simulink model "NeuromuscularModelwReflex2"  (R2019b)
settings: Solver=ode15s  StartTime=0.0  StopTime=30  MaxStep=.01  RelTol=1e-4  AbsTol=1e-6  EnableMultiTasking=on
values from neighbouring files (symbols this model uses):
  dt_visual = 1/30    (= 0.0333333333333)    [evaluateCost.m]    (also in optimize.m)
  LceOffsetTA = 1-0.5*w    [ControlParams.m]
  legAngleTgt = 1.2    [ControlParams.m]    (also in assignGains_novirtmuscle.m = Gains(38))
  LlegLengthClr = .9    (= 0.9)    [ControlParams.m]    (also in assignGains.m = Gains(39); assignGains_novirtmuscle.m = Gains(20))
  LongDelay = 0.020    (= 0.02)    [ControlParams.m]
  MidDelay = 0.010    (= 0.01)    [ControlParams.m]
  RlegLengthClr = .9    (= 0.9)    [ControlParams.m]    (also in assignGains.m = Gains(83); assignGains_novirtmuscle.m = Gains(34))
  ShortDelay = 0.005    [ControlParams.m]
  simbiconGainD = 5*pi/180    (= 0.0872664625997)    [ControlParams.m]    (also in assignGains_novirtmuscle.m = Gains(35))
  simbiconGainV = 5*pi/180    (= 0.0872664625997)    [ControlParams.m]    (also in assignGains_novirtmuscle.m = Gains(36))
  simbiconLegAngle0 = 85*pi/180    (= 1.4835298642)    [ControlParams.m]    (also in assignGains_novirtmuscle.m = Gains(37))
  termination_height = 0.5    [ControlParams.m]
undefined symbols (not defined in the file or in its folder): footCenterToCGDist, footInertia, footMass, g, loptGAS, loptHAM, loptHAMCut, loptTA, lslackGAS, lslackHAM, lslackHAMCut, phimaxGASa, phimaxGASk, phimaxHAMk, phirefGASa, phirefGASk, phirefHAMh, phirefHAMk, rGASa, rGASk, rHAMh, rHAMk, rhoGASa, rhoGASk, rhoHAMh, rhoHAMk, X, Y, Z
libraries: NeuroMuscularLibrary x88, sm_lib x22, nesl_utility x20, simulink x6, simulink_extras x2
(part 2 of 3)

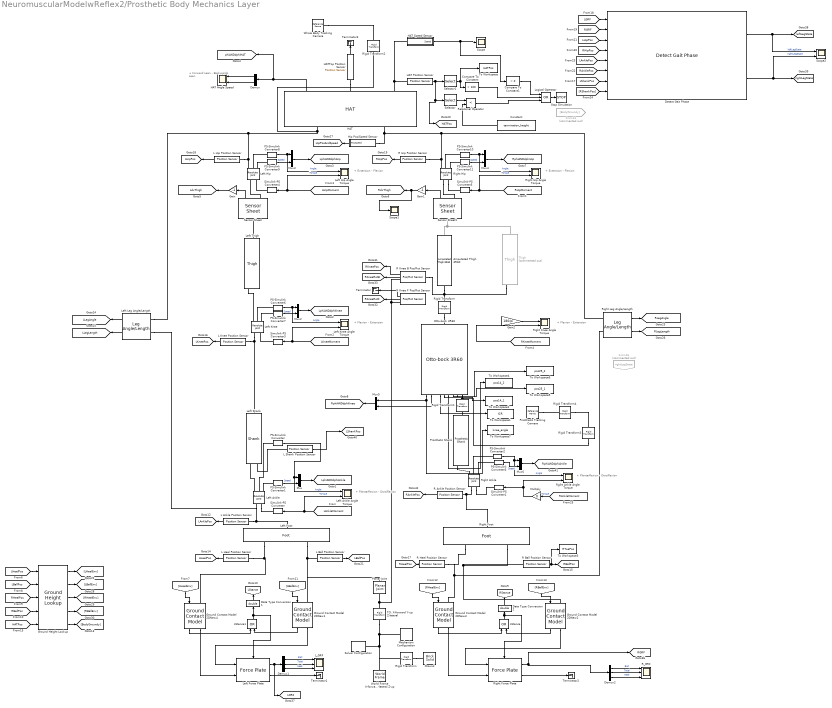
== system NeuromuscularModelwReflex2/Prosthetic Body Mechanics Layer ==
  note: + Plantarflexion
      | -  Dorsiflexion
  note: + Flexion
      | -  Extension
  note: + Extension
      | -  Flexion
  note: + Forward Lean
      | -  Backwards Lean
  note: + Extension
      | -  Flexion
  note: + Flexion
      | -  Extension
  note: + Plantarflexion
      | -  Dorsiflexion
  Amputated Thigh 3R60 : NeuroMuscularLibrary/Amputated Thigh 3R60  SystemSampleTime=-1  Latency=0  AutoFrameSizeCalculation=off
  Compare To Constant : simulink/Logic and Bit Operations/Compare To Constant  relop=>  const=100  OutDataTypeStr=boolean
  Compare To Constant1 : simulink/Logic and Bit Operations/Compare To Constant  relop=<  const=0  OutDataTypeStr=boolean
  Constant : Constant  Value=termination_height
  Data Type Conversion1 : DataTypeConversion  OutDataTypeStr=double
  Data Type Conversion2 : DataTypeConversion  OutDataTypeStr=double
  Demux : Demux  Outputs=2
  Demux1 : Demux  Outputs=3
  Demux2 : Demux  Outputs=3
  Detect Gait Phase : NeuroMuscularLibrary/Detect Gait Phase  SystemSampleTime=-1  Latency=0  AutoFrameSizeCalculation=off
  From14 : From  Commented=on  GotoTag=BodyGroundy
  From16 : From  Commented=on  GotoTag=rightLegState  TagVisibility=global
  Gain : Gain  Gain=-1
  Gain1 : Gain  Gain=-1
  Gain2 : Gain  Gain=180/pi
  Ground : sm_lib/Body Elements/Brick Solid  GraphicAmbientColor=[0.15 0.15 0.15 1.0]  BasedOnType=Density  BrickDimensions=[3 1 .01]  BrickDimensionUnits=m  CenterOfMass=[-footCenterToCGDist 0 0]  CenterOfMassUnits=m  GraphicDiffuseColor=[0.4 0.2 0.0]  Density=1000  DensityUnits=kg/(m^3)  DoExposeReferenceFrame=on  GraphicEmissiveColor=[0.0 0.0 0.0 1.0]  ExportEntireGeometry=off  SerializedFrames=<Frames/>  MarkerShape=Sphere  MarkerSize=10  GraphicType=FromGeometry  InertiaType=CalculateFromGeometry  Mass=footMass  MassUnits=kg  MomentsOfInertia=[0 0 footInertia]  MomentsOfInertiaUnits=kg*m^2  GraphicOpacity=1.0  ProductsOfInertia=[0 0 0]  ProductsOfInertiaUnits=kg*m^2  GraphicShininess=75  GraphicSpecularColor=[0.5 0.5 0.5 1.0]  GraphicVisPropType=SimpleVisualProperties
  Ground Contact Model 2DNew{1..4} (4 alike) : NeuroMuscularLibrary/Ground Contact Model  SystemSampleTime=-1  Latency=0  AutoFrameSizeCalculation=off
  Ground Height Lookup : NeuroMuscularLibrary/Ground Height Lookup  SystemSampleTime=-1  Latency=0  AutoFrameSizeCalculation=off
  HAT : NeuroMuscularLibrary/HAT  SystemSampleTime=-1  Latency=0  AutoFrameSizeCalculation=off
  HAT Position Sensor : NeuroMuscularLibrary/Position Sensor  SystemSampleTime=-1  Latency=0  AutoFrameSizeCalculation=off
  HAT Angle Speed : Scope  NumInputPorts=2
  HAT Speed Sensor : Subsystem
  HATTop Position Sensor : NeuroMuscularLibrary/Position Sensor  SystemSampleTime=-1  Latency=0  AutoFrameSizeCalculation=off
  Hip Pos/Speed Sensor : Subsystem
  L Ankle Position Sensor : NeuroMuscularLibrary/Position Sensor  SystemSampleTime=-1  Latency=0  AutoFrameSizeCalculation=off
  L Ball Position Sensor : NeuroMuscularLibrary/Position Sensor  SystemSampleTime=-1  Latency=0  AutoFrameSizeCalculation=off
  L Heel Position Sensor : NeuroMuscularLibrary/Position Sensor  SystemSampleTime=-1  Latency=0  AutoFrameSizeCalculation=off
  L Hip Position Sensor : NeuroMuscularLibrary/Position Sensor  SystemSampleTime=-1  Latency=0  AutoFrameSizeCalculation=off
  L Knee Position Sensor : NeuroMuscularLibrary/Position Sensor  SystemSampleTime=-1  Latency=0  AutoFrameSizeCalculation=off
  L Shank Position Sensor : NeuroMuscularLibrary/Position Sensor  SystemSampleTime=-1  Latency=0  AutoFrameSizeCalculation=off
  LStance : Logic  Operator=OR  AllPortsSameDT=off  OutDataTypeStr=boolean
  LStance1 : Logic  Operator=OR  AllPortsSameDT=off  OutDataTypeStr=boolean
  L_GRF : Scope  NumInputPorts=3
  Left Ankle : sm_lib/Joints/Revolute Joint  JointMode=Normal  SenseConstraintForce=off  SenseConstraintForceX=off  SenseConstraintForceY=off  SenseConstraintForceZ=off  SenseConstraintTorque=off  SenseConstraintTorqueX=off  SenseConstraintTorqueY=off  SenseConstraintTorqueZ=off  SenseTotalForce=off  SenseTotalForceX=off  SenseTotalForceY=off  SenseTotalForceZ=off  SenseTotalTorque=off  SenseTotalTorqueX=off  SenseTotalTorqueY=off  SenseTotalTorqueZ=off  CompositeWrenchDir=FollowerOnBase  CompositeWrenchFrame=BaseFrame  EquilibriumPosition=0  EquilibriumPositionUnits=deg  SpringStiffness=0  SpringStiffnessUnits=N*m/deg  DampingCoefficient=0  DampingCoefficientUnits=N*m/(deg/s)  TorqueActuationMode=InputTorque  MotionActuationMode=ComputedMotion  SensePosition=on  SenseVelocity=on  SenseAcceleration=off  SenseTorqueForce=off  SenseLowerLimitTorqueForce=off  SenseUpperLimitTorqueForce=off  LowerLimitSpecify=off  LowerLimitBound=-90  LowerLimitBoundUnits=deg  LowerLimitStiffness=1e4  LowerLimitStiffnessUnits=N*m/deg  LowerLimitDamping=10  LowerLimitDampingUnits=N*m/(deg/s)  LowerLimitTransitionRegionWidth=0.1  LowerLimitTransitionRegionWidthUnits=deg  UpperLimitSpecify=off  UpperLimitBound=90  UpperLimitBoundUnits=deg  UpperLimitStiffness=1e4  UpperLimitStiffnessUnits=N*m/deg  UpperLimitDamping=10  UpperLimitDampingUnits=N*m/(deg/s)  UpperLimitTransitionRegionWidth=0.1  UpperLimitTransitionRegionWidthUnits=deg  PositionTargetSpecify=on  PositionTargetPriority=High  PositionTargetValue=LphiAnkle0  PositionTargetValueUnits=rad  VelocityTargetSpecify=on  VelocityTargetPriority=Low  VelocityTargetValue=0  VelocityTargetValueUnits=rad/s
  Left Ankle Angle Torque : Scope  NumInputPorts=2
  Left Foot : NeuroMuscularLibrary/Foot  SystemSampleTime=-1  Latency=0  AutoFrameSizeCalculation=off
  Left Force Plate : NeuroMuscularLibrary/Force Plate  SystemSampleTime=-1  Latency=0  AutoFrameSizeCalculation=off
  Left Hip : sm_lib/Joints/Revolute Joint  JointMode=Normal  SenseConstraintForce=off  SenseConstraintForceX=off  SenseConstraintForceY=off  SenseConstraintForceZ=off  SenseConstraintTorque=off  SenseConstraintTorqueX=off  SenseConstraintTorqueY=off  SenseConstraintTorqueZ=off  SenseTotalForce=off  SenseTotalForceX=off  SenseTotalForceY=off  SenseTotalForceZ=off  SenseTotalTorque=off  SenseTotalTorqueX=off  SenseTotalTorqueY=off  SenseTotalTorqueZ=off  CompositeWrenchDir=FollowerOnBase  CompositeWrenchFrame=BaseFrame  EquilibriumPosition=0  EquilibriumPositionUnits=deg  SpringStiffness=0  SpringStiffnessUnits=N*m/deg  DampingCoefficient=0  DampingCoefficientUnits=N*m/(deg/s)  TorqueActuationMode=InputTorque  MotionActuationMode=ComputedMotion  SensePosition=on  SenseVelocity=on  SenseAcceleration=off  SenseTorqueForce=off  SenseLowerLimitTorqueForce=off  SenseUpperLimitTorqueForce=off  LowerLimitSpecify=off  LowerLimitBound=-90  LowerLimitBoundUnits=deg  LowerLimitStiffness=1e4  LowerLimitStiffnessUnits=N*m/deg  LowerLimitDamping=10  LowerLimitDampingUnits=N*m/(deg/s)  LowerLimitTransitionRegionWidth=0.1  LowerLimitTransitionRegionWidthUnits=deg  UpperLimitSpecify=off  UpperLimitBound=90  UpperLimitBoundUnits=deg  UpperLimitStiffness=1e4  UpperLimitStiffnessUnits=N*m/deg  UpperLimitDamping=10  UpperLimitDampingUnits=N*m/(deg/s)  UpperLimitTransitionRegionWidth=0.1  UpperLimitTransitionRegionWidthUnits=deg  PositionTargetSpecify=on  PositionTargetPriority=High  PositionTargetValue=LphiHip0  PositionTargetValueUnits=rad  VelocityTargetSpecify=on  VelocityTargetPriority=Low  VelocityTargetValue=0  VelocityTargetValueUnits=deg/s
  Left Hip Angle Torque : Scope  NumInputPorts=2
  Left Knee : sm_lib/Joints/Revolute Joint  JointMode=Normal  SenseConstraintForce=off  SenseConstraintForceX=off  SenseConstraintForceY=off  SenseConstraintForceZ=off  SenseConstraintTorque=off  SenseConstraintTorqueX=off  SenseConstraintTorqueY=off  SenseConstraintTorqueZ=off  SenseTotalForce=off  SenseTotalForceX=off  SenseTotalForceY=off  SenseTotalForceZ=off  SenseTotalTorque=off  SenseTotalTorqueX=off  SenseTotalTorqueY=off  SenseTotalTorqueZ=off  CompositeWrenchDir=FollowerOnBase  CompositeWrenchFrame=BaseFrame  EquilibriumPosition=0  EquilibriumPositionUnits=deg  SpringStiffness=0  SpringStiffnessUnits=N*m/deg  DampingCoefficient=0  DampingCoefficientUnits=N*m/(deg/s)  TorqueActuationMode=InputTorque  MotionActuationMode=ComputedMotion  SensePosition=on  SenseVelocity=on  SenseAcceleration=off  SenseTorqueForce=off  SenseLowerLimitTorqueForce=off  SenseUpperLimitTorqueForce=off  LowerLimitSpecify=off  LowerLimitBound=-90  LowerLimitBoundUnits=deg  LowerLimitStiffness=1e4  LowerLimitStiffnessUnits=N*m/deg  LowerLimitDamping=10  LowerLimitDampingUnits=N*m/(deg/s)  LowerLimitTransitionRegionWidth=0.1  LowerLimitTransitionRegionWidthUnits=deg  UpperLimitSpecify=off  UpperLimitBound=90  UpperLimitBoundUnits=deg  UpperLimitStiffness=1e4  UpperLimitStiffnessUnits=N*m/deg  UpperLimitDamping=10  UpperLimitDampingUnits=N*m/(deg/s)  UpperLimitTransitionRegionWidth=0.1  UpperLimitTransitionRegionWidthUnits=deg  PositionTargetSpecify=on  PositionTargetPriority=High  PositionTargetValue=LphiKnee0  PositionTargetValueUnits=rad  VelocityTargetSpecify=on  VelocityTargetPriority=Low  VelocityTargetValue=0  VelocityTargetValueUnits=deg/s
  Left Knee Angle Torque : Scope  NumInputPorts=2
  Left Leg Angle/Length : NeuroMuscularLibrary/Leg Angle//Length  SystemSampleTime=-1  Latency=0  AutoFrameSizeCalculation=off
  Left Shank : NeuroMuscularLibrary/Shank  SystemSampleTime=-1  Latency=0  AutoFrameSizeCalculation=off
  Left Thigh : NeuroMuscularLibrary/Thigh  SystemSampleTime=-1  Latency=0  AutoFrameSizeCalculation=off
  Logical Operator : Logic  Operator=OR  Inputs=3  AllPortsSameDT=off  OutDataTypeStr=boolean
  Mechanism Configuration : sm_lib/Utilities/Mechanism Configuration  UniformGravity=Constant  GravityVector=[0 0 -g]  GravityUnits=m/s^2  LinearizationDelta=0.001
  Multiply : Gain  Gain=0
  Mux{,2..6} (6 alike) : Mux  Inputs=2
  Otto-bock 3R60 : NeuroMuscularLibrary/Otto-bock 3R60  SystemSampleTime=-1  Latency=0  AutoFrameSizeCalculation=off
  PS-Simulink Converter{,2,6,8,10} (5 alike) : nesl_utility/PS-Simulink Converter  PhysicalDomain=network_engine_domain  SubClassName=ps_output  LeftPortType=input  RightPortType=output  PseudoPeriodic=off  Frequencies=[]  Unit=rad  AffineConversion=off
  PS-Simulink Converter{1,3,7,9,11} (5 alike) : nesl_utility/PS-Simulink Converter  PhysicalDomain=network_engine_domain  SubClassName=ps_output  LeftPortType=input  RightPortType=output  PseudoPeriodic=off  Frequencies=[]  Unit=rad/s  AffineConversion=off
  Planar Joint : sm_lib/Joints/Planar Joint  JointMode=Normal  SenseConstraintForce=off  SenseConstraintForceX=off  SenseConstraintForceY=off  SenseConstraintForceZ=off  SenseConstraintTorque=off  SenseConstraintTorqueX=off  SenseConstraintTorqueY=off  SenseConstraintTorqueZ=off  SenseTotalForce=off  SenseTotalForceX=off  SenseTotalForceY=off  SenseTotalForceZ=off  SenseTotalTorque=off  SenseTotalTorqueX=off  SenseTotalTorqueY=off  SenseTotalTorqueZ=off  CompositeWrenchDir=FollowerOnBase  CompositeWrenchFrame=BaseFrame  PxEquilibriumPosition=0  PxEquilibriumPositionUnits=m  PxSpringStiffness=0  PxSpringStiffnessUnits=N/m  PxDampingCoefficient=0  PxDampingCoefficientUnits=N/(m/s)  PxTorqueActuationMode=NoTorque  PxMotionActuationMode=ComputedMotion  PxSensePosition=off  PxSenseVelocity=off  PxSenseAcceleration=off  PxSenseTorqueForce=off  PxSenseLowerLimitTorqueForce=off  PxSenseUpperLimitTorqueForce=off  PxLowerLimitSpecify=off  PxLowerLimitBound=-1  PxLowerLimitBoundUnits=m  PxLowerLimitStiffness=1e6  PxLowerLimitStiffnessUnits=N/m  PxLowerLimitDamping=1e3  PxLowerLimitDampingUnits=N/(m/s)  PxLowerLimitTransitionRegionWidth=1e-4  PxLowerLimitTransitionRegionWidthUnits=m  PxUpperLimitSpecify=off  PxUpperLimitBound=1  PxUpperLimitBoundUnits=m  PxUpperLimitStiffness=1e6  PxUpperLimitStiffnessUnits=N/m  PxUpperLimitDamping=1e3  PxUpperLimitDampingUnits=N/(m/s)  PxUpperLimitTransitionRegionWidth=1e-4  PxUpperLimitTransitionRegionWidthUnits=m  PxPositionTargetSpecify=on  PxPositionTargetPriority=Low  PxPositionTargetValue=0  PxPositionTargetValueUnits=m  PxVelocityTargetSpecify=on  PxVelocityTargetPriority=High  PxVelocityTargetValue=vx0  PxVelocityTargetValueUnits=m/s  PyEquilibriumPosition=0  PyEquilibriumPositionUnits=m  PySpringStiffness=0  PySpringStiffnessUnits=N/m  PyDampingCoefficient=0  PyDampingCoefficientUnits=N/(m/s)  PyTorqueActuationMode=NoTorque  PyMotionActuationMode=ComputedMotion  PySensePosition=off  PySenseVelocity=off  PySenseAcceleration=off  PySenseTorqueForce=off  PySenseLowerLimitTorqueForce=off  PySenseUpperLimitTorqueForce=off  PyLowerLimitSpecify=off  PyLowerLimitBound=-1  PyLowerLimitBoundUnits=m  PyLowerLimitStiffness=1e6  PyLowerLimitStiffnessUnits=N/m  PyLowerLimitDamping=1e3  PyLowerLimitDampingUnits=N/(m/s)  PyLowerLimitTransitionRegionWidth=1e-4  PyLowerLimitTransitionRegionWidthUnits=m  PyUpperLimitSpecify=off  PyUpperLimitBound=1  PyUpperLimitBoundUnits=m  PyUpperLimitStiffness=1e6  PyUpperLimitStiffnessUnits=N/m  PyUpperLimitDamping=1e3  PyUpperLimitDampingUnits=N/(m/s)  PyUpperLimitTransitionRegionWidth=1e-4  PyUpperLimitTransitionRegionWidthUnits=m  PyPositionTargetSpecify=on  PyPositionTargetPriority=Low  PyPositionTargetValue=0  PyPositionTargetValueUnits=m  PyVelocityTargetSpecify=on  PyVelocityTargetPriority=Low  PyVelocityTargetValue=0  PyVelocityTargetValueUnits=m/s  RzEquilibriumPosition=0  RzEquilibriumPositionUnits=deg  RzSpringStiffness=0  RzSpringStiffnessUnits=N*m/deg  RzDampingCoefficient=0  RzDampingCoefficientUnits=N*m/(deg/s)  RzTorqueActuationMode=NoTorque  RzMotionActuationMode=ComputedMotion  RzSensePosition=off  RzSenseVelocity=off  RzSenseAcceleration=off  RzSenseTorqueForce=off  RzSenseLowerLimitTorqueForce=off  RzSenseUpperLimitTorqueForce=off  RzLowerLimitSpecify=off  RzLowerLimitBound=-90  RzLowerLimitBoundUnits=deg  RzLowerLimitStiffness=1e4  RzLowerLimitStiffnessUnits=N*m/deg  RzLowerLimitDamping=10  RzLowerLimitDampingUnits=N*m/(deg/s)  RzLowerLimitTransitionRegionWidth=0.1  RzLowerLimitTransitionRegionWidthUnits=deg  RzUpperLimitSpecify=off  RzUpperLimitBound=90  RzUpperLimitBoundUnits=deg  RzUpperLimitStiffness=1e4  RzUpperLimitStiffnessUnits=N*m/deg  RzUpperLimitDamping=10  RzUpperLimitDampingUnits=N*m/(deg/s)  RzUpperLimitTransitionRegionWidth=0.1  RzUpperLimitTransitionRegionWidthUnits=deg  RzPositionTargetSpecify=on  RzPositionTargetPriority=Low  RzPositionTargetValue=0  RzPositionTargetValueUnits=deg  RzVelocityTargetSpecify=on  RzVelocityTargetPriority=Low  RzVelocityTargetValue=0  RzVelocityTargetValueUnits=deg/s
  Prosthesis Tracking Camera : sm_lib/Frames and Transforms/Reference Frame
  Prosthetic Shank : NeuroMuscularLibrary/Prosthetic Shank  SystemSampleTime=-1  Latency=0  AutoFrameSizeCalculation=off
  R Ankle Position Sensor : NeuroMuscularLibrary/Position Sensor  SystemSampleTime=-1  Latency=0  AutoFrameSizeCalculation=off
  R Ball Position Sensor : NeuroMuscularLibrary/Position Sensor  SystemSampleTime=-1  Latency=0  AutoFrameSizeCalculation=off
  R Heel Position Sensor : NeuroMuscularLibrary/Position Sensor  SystemSampleTime=-1  Latency=0  AutoFrameSizeCalculation=off
  R Hip Position Sensor : NeuroMuscularLibrary/Position Sensor  SystemSampleTime=-1  Latency=0  AutoFrameSizeCalculation=off
  R Knee B Pos/Rot Sensor : NeuroMuscularLibrary/Pos//Rot Sensor  SystemSampleTime=-1  Latency=0  AutoFrameSizeCalculation=off
  R Knee F Pos/Rot Sensor : NeuroMuscularLibrary/Pos//Rot Sensor  SystemSampleTime=-1  Latency=0  AutoFrameSizeCalculation=off
  R_GRF : Scope  NumInputPorts=3
  Relational Operator : RelationalOperator  Operator=<  OutDataTypeStr=boolean  RndMeth=Nearest
  Rgiht Ankle Angle Torque : Scope  NumInputPorts=2
  Right Ankle : sm_lib/Joints/Revolute Joint  JointMode=Normal  SenseConstraintForce=off  SenseConstraintForceX=off  SenseConstraintForceY=off  SenseConstraintForceZ=off  SenseConstraintTorque=off  SenseConstraintTorqueX=off  SenseConstraintTorqueY=off  SenseConstraintTorqueZ=off  SenseTotalForce=off  SenseTotalForceX=off  SenseTotalForceY=off  SenseTotalForceZ=off  SenseTotalTorque=off  SenseTotalTorqueX=off  SenseTotalTorqueY=off  SenseTotalTorqueZ=off  CompositeWrenchDir=FollowerOnBase  CompositeWrenchFrame=BaseFrame  EquilibriumPosition=0  EquilibriumPositionUnits=deg  SpringStiffness=20  SpringStiffnessUnits=N*m/deg  DampingCoefficient=4  DampingCoefficientUnits=N*m/(deg/s)  TorqueActuationMode=InputTorque  MotionActuationMode=ComputedMotion  SensePosition=on  SenseVelocity=on  SenseAcceleration=off  SenseTorqueForce=off  SenseLowerLimitTorqueForce=off  SenseUpperLimitTorqueForce=off  LowerLimitSpecify=off  LowerLimitBound=-90  LowerLimitBoundUnits=deg  LowerLimitStiffness=1e4  LowerLimitStiffnessUnits=N*m/deg  LowerLimitDamping=10  LowerLimitDampingUnits=N*m/(deg/s)  LowerLimitTransitionRegionWidth=0.1  LowerLimitTransitionRegionWidthUnits=deg  UpperLimitSpecify=off  UpperLimitBound=90  UpperLimitBoundUnits=deg  UpperLimitStiffness=1e4  UpperLimitStiffnessUnits=N*m/deg  UpperLimitDamping=10  UpperLimitDampingUnits=N*m/(deg/s)  UpperLimitTransitionRegionWidth=0.1  UpperLimitTransitionRegionWidthUnits=deg  PositionTargetSpecify=on  PositionTargetPriority=High  PositionTargetValue=RphiAnkle0  PositionTargetValueUnits=rad  VelocityTargetSpecify=on  VelocityTargetPriority=Low  VelocityTargetValue=0  VelocityTargetValueUnits=rad/s
  Right Foot : NeuroMuscularLibrary/Foot  SystemSampleTime=-1  Latency=0  AutoFrameSizeCalculation=off
      link override Foot Solid: Mass=1  MomentsOfInertia=[0 0 0]
  Right Force Plate : NeuroMuscularLibrary/Force Plate  SystemSampleTime=-1  Latency=0  AutoFrameSizeCalculation=off
  Right Hip : sm_lib/Joints/Revolute Joint  JointMode=Normal  SenseConstraintForce=off  SenseConstraintForceX=off  SenseConstraintForceY=off  SenseConstraintForceZ=off  SenseConstraintTorque=off  SenseConstraintTorqueX=off  SenseConstraintTorqueY=off  SenseConstraintTorqueZ=off  SenseTotalForce=off  SenseTotalForceX=off  SenseTotalForceY=off  SenseTotalForceZ=off  SenseTotalTorque=off  SenseTotalTorqueX=off  SenseTotalTorqueY=off  SenseTotalTorqueZ=off  CompositeWrenchDir=FollowerOnBase  CompositeWrenchFrame=BaseFrame  EquilibriumPosition=0  EquilibriumPositionUnits=deg  SpringStiffness=0  SpringStiffnessUnits=N*m/deg  DampingCoefficient=0  DampingCoefficientUnits=N*m/(deg/s)  TorqueActuationMode=InputTorque  MotionActuationMode=ComputedMotion  SensePosition=on  SenseVelocity=on  SenseAcceleration=off  SenseTorqueForce=off  SenseLowerLimitTorqueForce=off  SenseUpperLimitTorqueForce=off  LowerLimitSpecify=off  LowerLimitBound=-90  LowerLimitBoundUnits=deg  LowerLimitStiffness=1e4  LowerLimitStiffnessUnits=N*m/deg  LowerLimitDamping=10  LowerLimitDampingUnits=N*m/(deg/s)  LowerLimitTransitionRegionWidth=0.1  LowerLimitTransitionRegionWidthUnits=deg  UpperLimitSpecify=off  UpperLimitBound=90  UpperLimitBoundUnits=deg  UpperLimitStiffness=1e4  UpperLimitStiffnessUnits=N*m/deg  UpperLimitDamping=10  UpperLimitDampingUnits=N*m/(deg/s)  UpperLimitTransitionRegionWidth=0.1  UpperLimitTransitionRegionWidthUnits=deg  PositionTargetSpecify=on  PositionTargetPriority=High  PositionTargetValue=RphiHip0  PositionTargetValueUnits=rad  VelocityTargetSpecify=on  VelocityTargetPriority=Low  VelocityTargetValue=0  VelocityTargetValueUnits=deg/s
  Right Hip Angle Torque : Scope  NumInputPorts=2
  Right Knee Angle Torque : Scope  NumInputPorts=2
  Right Leg Angle/Length : NeuroMuscularLibrary/Leg Angle//Length  SystemSampleTime=-1  Latency=0  AutoFrameSizeCalculation=off
  Rigid Transform : sm_lib/Frames and Transforms/Rigid Transform  TranslationMethod=None  TranslationStandardOffset=0  TranslationLengthUnit=m  TranslationStandardAxis=+Z  TranslationCartesianOffset=[0 0 0]  TranslationROffset=0  TranslationROffsetUnits=m  TranslationZOffset=0  TranslationZOffsetUnits=m  TranslationThetaOffset=0  TranslationThetaOffsetUnits=deg  RotationMethod=AlignedAxes  RotationAngleUnits=deg  RotationStandardAxis=+Z  RotationAngle=0.0  RotationArbitraryAxis=[0 0 1]  FollAlignAxisA=+Z  BaseAlignAxisA=-Z  FollAlignAxisB=+Y  BaseAlignAxisB=+X  RotationSequenceAxes=FollowerAxes  RotationSequence=XYX  RotationSequenceAngles=[0 0 0]  RotationSequenceAnglesUnits=deg  RotationMatrix=[1 0 0; 0 1 0; 0 0 1]
  Rigid Transform1 : sm_lib/Frames and Transforms/Rigid Transform  TranslationMethod=None  TranslationStandardOffset=0  TranslationLengthUnit=m  TranslationStandardAxis=+Z  TranslationCartesianOffset=[0 0 0]  TranslationROffset=0  TranslationROffsetUnits=m  TranslationZOffset=0  TranslationZOffsetUnits=m  TranslationThetaOffset=0  TranslationThetaOffsetUnits=deg  RotationMethod=AlignedAxes  RotationAngleUnits=deg  RotationStandardAxis=+Z  RotationAngle=0.0  RotationArbitraryAxis=[0 0 1]  FollAlignAxisA=+Z  BaseAlignAxisA=-Z  FollAlignAxisB=+Y  BaseAlignAxisB=+X  RotationSequenceAxes=FollowerAxes  RotationSequence=XYX  RotationSequenceAngles=[0 0 0]  RotationSequenceAnglesUnits=deg  RotationMatrix=[1 0 0; 0 1 0; 0 0 1]
  Rigid Transform2 : sm_lib/Frames and Transforms/Rigid Transform  TranslationMethod=StandardAxis  TranslationStandardOffset=3  TranslationLengthUnit=m  TranslationStandardAxis=+Z  TranslationCartesianOffset=[0 0 0]  TranslationROffset=0  TranslationROffsetUnits=m  TranslationZOffset=0  TranslationZOffsetUnits=m  TranslationThetaOffset=0  TranslationThetaOffsetUnits=deg  RotationMethod=None  RotationAngleUnits=deg  RotationStandardAxis=+Z  RotationAngle=0.0  RotationArbitraryAxis=[0 0 1]  FollAlignAxisA=+X  BaseAlignAxisA=+Y  FollAlignAxisB=+Y  BaseAlignAxisB=+Z  RotationSequenceAxes=FollowerAxes  RotationSequence=XYX  RotationSequenceAngles=[0 0 0]  RotationSequenceAnglesUnits=deg  RotationMatrix=[1 0 0; 0 1 0; 0 0 1]
  Rigid Transform3 : sm_lib/Frames and Transforms/Rigid Transform  TranslationMethod=StandardAxis  TranslationStandardOffset=0.5  TranslationLengthUnit=m  TranslationStandardAxis=-Z  TranslationCartesianOffset=[0 0 0]  TranslationROffset=0  TranslationROffsetUnits=m  TranslationZOffset=0  TranslationZOffsetUnits=m  TranslationThetaOffset=0  TranslationThetaOffsetUnits=deg  RotationMethod=None  RotationAngleUnits=deg  RotationStandardAxis=+Z  RotationAngle=0.0  RotationArbitraryAxis=[0 0 1]  FollAlignAxisA=+X  BaseAlignAxisA=+Y  FollAlignAxisB=+Y  BaseAlignAxisB=+Z  RotationSequenceAxes=FollowerAxes  RotationSequence=XYX  RotationSequenceAngles=[0 0 0]  RotationSequenceAnglesUnits=deg  RotationMatrix=[1 0 0; 0 1 0; 0 0 1]
  Rigid Transform4 : sm_lib/Frames and Transforms/Rigid Transform  TranslationMethod=StandardAxis  TranslationStandardOffset=0.5  TranslationLengthUnit=m  TranslationStandardAxis=-Z  TranslationCartesianOffset=[0 0 0]  TranslationROffset=0  TranslationROffsetUnits=m  TranslationZOffset=0  TranslationZOffsetUnits=m  TranslationThetaOffset=0  TranslationThetaOffsetUnits=deg  RotationMethod=None  RotationAngleUnits=deg  RotationStandardAxis=+Z  RotationAngle=0.0  RotationArbitraryAxis=[0 0 1]  FollAlignAxisA=+X  BaseAlignAxisA=+Y  FollAlignAxisB=+Y  BaseAlignAxisB=+Z  RotationSequenceAxes=FollowerAxes  RotationSequence=XYX  RotationSequenceAngles=[0 0 0]  RotationSequenceAnglesUnits=deg  RotationMatrix=[1 0 0; 0 1 0; 0 0 1]
  Rigid Transform : sm_lib/Frames and Transforms/Rigid Transform  TranslationMethod=Cartesian  TranslationStandardOffset=1  TranslationLengthUnit=m  TranslationStandardAxis=+X  TranslationCartesianOffset="[1  0 0]"  TranslationROffset=0  TranslationROffsetUnits=m  TranslationZOffset=0  TranslationZOffsetUnits=m  TranslationThetaOffset=0  TranslationThetaOffsetUnits=deg  RotationMethod=None  RotationAngleUnits=deg  RotationStandardAxis=+Z  RotationAngle=0  RotationArbitraryAxis=[0 0 1]  FollAlignAxisA=+X  BaseAlignAxisA=+Y  FollAlignAxisB=+Y  BaseAlignAxisB=+Z  RotationSequenceAxes=FollowerAxes  RotationSequence=XYX  RotationSequenceAngles=[0 0 0]  RotationSequenceAnglesUnits=deg  RotationMatrix=[1 0 0; 0 1 0; 0 0 1]
  Scope : Scope
  Scope1 : Scope
  Scope2 : Scope  NumInputPorts=2
  Selector : Selector  InputPortWidth=3  IndexOptions=Index vector (dialog)  Indices=[3]  OutputSizes=1
  Selector1 : Selector  InputPortWidth=3  IndexOptions=Index vector (dialog)  Indices=[1]  OutputSizes=1
  Sensor Sheet : NeuroMuscularLibrary/Sensor Sheet  SystemSampleTime=-1  Latency=0  AutoFrameSizeCalculation=off
  Sensor Sheet1 : NeuroMuscularLibrary/Sensor Sheet  SystemSampleTime=-1  Latency=0  AutoFrameSizeCalculation=off
  Simulink-PS Converter{,1,3..5} (5 alike) : nesl_utility/Simulink-PS Converter  PhysicalDomain=network_engine_domain  SubClassName=ps_input  LeftPortType=input  RightPortType=output  PseudoPeriodic=off  Frequencies=[]  NoiseDistribution=none  NoiseParameters=[]  Unit=N*m  AffineConversion=off  FilteringAndDerivatives=zero  SimscapeFilterOrder=1  InputFilterTimeConstant=0.001  UdotUserProvided=1
  Solver Configuration : nesl_utility/Solver Configuration  PhysicalDomain=network_engine_domain  SubClassName=solver  LeftPortType=input  RightPortType=generic  Tones=[]  Harmonics=[]  SimulateNoise=off  Profile=off  UseLocalSampling=off  EnableSwitchedLinearOptims=on  FrequencyDomain=off  UseCCode=off  RelTol=0.001  AbsTol=1e-06  MinStep=1e-09  ToWorkspace=off  RevertToSquareIcSolve=off  NumHomotopyIterations=100  PhasorMode=off  PhasorModeNumHarmonics=1  DoDC=off  ResidualTolerance=1e-09  UseLocalSolver=off  LocalSolverChoice=NE_BACKWARD_EULER_ADVANCER  LocalSolverSampleTime=0.001  DoFixedCost=off  MaxNonlinIter=3  MaxModeIter=2  LinearAlgebra=Sparse  EquationFormulation=NE_TIME_EF  DelaysMemoryBudget=1024  AutomaticFiltering=on  FilteringTimeConstant=0.001  PartitionStorageMethod=AS_NEEDED  PartitionMemoryBudget=1024  PartitionMethod=FAST
  Stop Simulation : Stop
  TO: X-forward Y-up Z-lateral : sm_lib/Frames and Transforms/Rigid Transform  TranslationMethod=StandardAxis  TranslationStandardOffset=hatLeftHipToCenterDistWidth  TranslationLengthUnit=m  TranslationStandardAxis=+Z  TranslationCartesianOffset=[0 0 0]  TranslationROffset=0  TranslationROffsetUnits=m  TranslationZOffset=0  TranslationZOffsetUnits=m  TranslationThetaOffset=0  TranslationThetaOffsetUnits=deg  RotationMethod=AlignedAxes  RotationAngleUnits=deg  RotationStandardAxis=+Z  RotationAngle=0  RotationArbitraryAxis=[0 0 1]  FollAlignAxisA=+Z  BaseAlignAxisA=+Y  FollAlignAxisB=+X  BaseAlignAxisB=+X  RotationSequenceAxes=FollowerAxes  RotationSequence=XYX  RotationSequenceAngles=[0 0 0]  RotationSequenceAnglesUnits=deg  RotationMatrix=[1 0 0; 0 1 0; 0 0 1]
  Terminator{,1..3} (4 alike) : Terminator
  Thigh : NeuroMuscularLibrary/Thigh  Commented=on  SystemSampleTime=-1  Latency=0  AutoFrameSizeCalculation=off
  To Workspace : ToWorkspace  VariableName=HATPos  SampleTime=-1
      settings: MaxDataPoints=1
  To Workspace1 : ToWorkspace  VariableName=ICR  SampleTime=dt_visual
  To Workspace2 : ToWorkspace  VariableName=pos14_1  SampleTime=dt_visual
  To Workspace3 : ToWorkspace  VariableName=RToePos  SaveFormat=Structure With Time  SampleTime=-1
  To Workspace4 : ToWorkspace  VariableName=pos14_2  SampleTime=dt_visual
  To Workspace5 : ToWorkspace  VariableName=pos25_1  SampleTime=dt_visual
  To Workspace6 : ToWorkspace  VariableName=pos25_2  SampleTime=dt_visual
  To Workspace7 : ToWorkspace  VariableName=knee_angle  SampleTime=dt_visual
  Whole Body Tracking Camera : sm_lib/Frames and Transforms/Reference Frame
  World Frame X-forward Y-lateral Z-up : sm_lib/Frames and Transforms/World Frame
  tag scope: HATPos=global, HipPosAndSpeed=global, LAnklePos=global, LBallPos=global, LGRF=global, LHeelPos=global, LHipPos=global, LKneePos=global, LLegAngle=global, LLegLength=global, LShankPos=global, LStance=global, LdxThigh=global, LphiANDdphiAnkle=global, LphiANDdphiHip=global, LphiANDdphiKnee=global, RAnklePos=global, RBallPos=global, RGRF=global, RHeelPos=global, RHipPos=global, RKneePos=global, RKneeRotB=global, RKneeRotF=global, RLegAngle=global, RLegLength=global, RStance=global, RdxThigh=global, RphiANDdphiAnkle=global, RphiANDdphiHip=global, RphiANDdphiKnee=global, leftLegState=global, phiANDdphiHAT=global, rightLegState=global
  wires:
  Left Force Plate/1 -> [LGRF], Demux1/1
  Demux1/1 -> L_GRF/1  "Ball"
  Demux1/2 -> L_GRF/2  "Total"
  Demux1/3 -> L_GRF/3  "Heel"
  Left Force Plate/2 -> Terminator1/1
  Ground Contact Model 2DNew1/2 -> Left Force Plate/1
  Ground Contact Model 2DNew4/2 -> Left Force Plate/2
  Right Force Plate/1 -> [RGRF], Demux2/1
  Demux2/1 -> R_GRF/1  "Ball"
  Demux2/2 -> R_GRF/2  "Total"
  Demux2/3 -> R_GRF/3  "Heel"
  Right Force Plate/2 -> Terminator2/1
  Ground Contact Model 2DNew2/2 -> Right Force Plate/1
  Ground Contact Model 2DNew3/2 -> Right Force Plate/2
  LStance/1 -> Right Force Plate/Enable, Data Type Conversion2/1
  Mux/1 -> [LphiANDdphiAnkle]
  PS-Simulink Converter6/1 -> Left Knee Angle Torque/1, Mux2/1  "Angle"
  PS-Simulink Converter7/1 -> Mux2/2  "Speed"
  Demux/1 -> HAT Angle Speed/1
  PS-Simulink Converter/1 -> Left Ankle Angle Torque/1, Mux/1  "Angle"
  PS-Simulink Converter1/1 -> Mux/2  "Speed"
  Mux2/1 -> [LphiANDdphiKnee]
  [LKneeMoment] -> Simulink-PS Converter3/1, Left Knee Angle Torque/2
  Sensor Sheet/1 -> Gain/1
  PS-Simulink Converter9/1 -> Mux3/2  "Speed"
  HAT/1 -> [phiANDdphiHAT], Demux/1
  Demux/2 -> HAT Angle Speed/2
  Mux3/1 -> [LphiANDdphiHip]
  Gain/1 -> [LdxThigh]
  Sensor Sheet1/1 -> Gain1/1
  Gain1/1 -> Scope1/1, [RdxThigh]
  Ground Contact Model 2DNew3/1 -> LStance/1
  Ground Contact Model 2DNew2/1 -> LStance/2
  LStance1/1 -> Left Force Plate/Enable, Data Type Conversion1/1
  Ground Contact Model 2DNew4/1 -> LStance1/1
  Ground Contact Model 2DNew1/1 -> LStance1/2
  Mux5/1 -> [RphiANDdphiKnee]
  Mux4/1 -> [RphiANDdphiHip]
  L Ankle Position Sensor/1 -> [LAnklePos]
  L Heel Position Sensor/1 -> [LHeelPos]
  L Knee Position Sensor/1 -> [LKneePos]
  L Hip Position Sensor/1 -> [LHipPos]
  R Hip Position Sensor/1 -> [RHipPos]
  L Ball Position Sensor/1 -> [LBallPos]
  [RKneeMoment] -> Right Knee Angle Torque/2
  [LAnkleMoment] -> Simulink-PS Converter/1, Left Ankle Angle Torque/2  "Torque"
  [LHipMoment] -> Left Hip Angle Torque/2, Simulink-PS Converter4/1  "Torque"
  PS-Simulink Converter8/1 -> Left Hip Angle Torque/1, Mux3/1  "Angle"
  [RHipMoment] -> Right Hip Angle Torque/2, Simulink-PS Converter5/1  "Torque"
  PS-Simulink Converter10/1 -> Right Hip Angle Torque/1, Mux4/1  "Angle"
  PS-Simulink Converter11/1 -> Mux4/2  "Speed"
  Selector/1 -> Relational Operator/1
  Selector1/1 -> Compare To Constant/1, To Workspace/1
  Hip Pos/Speed Sensor/1(PosSpeed) -> [HipPosAndSpeed]
  Right Leg Angle/Length/1 -> [RLegAngle]
  Right Leg Angle/Length/2 -> [RLegLength]
  Left Leg Angle/Length/1 -> [LLegAngle]
  Left Leg Angle/Length/2 -> [LLegLength]
  Data Type Conversion1/1 -> [LStance]
  Data Type Conversion2/1 -> [RStance]
  R Ball Position Sensor/1 -> To Workspace3/1, [RBallPos]
  R Heel Position Sensor/1 -> [RHeelPos]
  [LHeelEnv] -> Ground Contact Model 2DNew4/1
  [LBallEnv] -> Ground Contact Model 2DNew1/1
  [RHeelEnv] -> Ground Contact Model 2DNew3/1
  [RBallEnv] -> Ground Contact Model 2DNew2/1
  R Knee F Pos/Rot Sensor/2 -> [RKneeRotF]
  R Knee B Pos/Rot Sensor/2 -> [RKneeRotB]
  R Knee B Pos/Rot Sensor/1 -> [RKneePos]
  HAT Position Sensor/1 -> [HATPos], Selector/1, Selector1/1
  Compare To Constant/1 -> Logical Operator/2
  R Knee F Pos/Rot Sensor/1 -> Terminator/1
  Relational Operator/1 -> Logical Operator/3
  Logical Operator/1 -> Stop Simulation/1
  HATTop Position Sensor/1 -> Terminator3/1
  HAT Speed Sensor/1(Speed) -> Compare To Constant1/1, Scope/1
  [LHeelPos] -> Ground Height Lookup/1
  Ground Height Lookup/1 -> [LHeelEnv]
  [LBallPos] -> Ground Height Lookup/2
  Ground Height Lookup/2 -> [LBallEnv]
  [RHeelPos] -> Ground Height Lookup/3
  Ground Height Lookup/3 -> [RHeelEnv]
  Ground Height Lookup/4 -> [RBallEnv]
  Ground Height Lookup/5 -> [BodyGroundy]
  [HATPos] -> Ground Height Lookup/5
  Gain2/1 -> Right Knee Angle Torque/1
  [RBallPos] -> Ground Height Lookup/4
  [RHipPos] -> Detect Gait Phase/4
  [LAnklePos] -> Detect Gait Phase/5
  Detect Gait Phase/2 -> Scope2/2, [rightLegState]  "rightLegState"
  [RGRF] -> Detect Gait Phase/2
  [RShankPos] -> Detect Gait Phase/8
  [LHipPos] -> Detect Gait Phase/3
  [LShankPos] -> Detect Gait Phase/7
  [LGRF] -> Detect Gait Phase/1
  Detect Gait Phase/1 -> Scope2/1, [leftLegState]  "leftLegState"
  [RAnklePos] -> Detect Gait Phase/6
  L Shank Position Sensor/1 -> [LShankPos]
  Constant/1 -> Relational Operator/2
  Compare To Constant1/1 -> Logical Operator/1
  PS-Simulink Converter3/1 -> Mux6/2  "Speed"
  R Ankle Position Sensor/1 -> [RAnklePos]
  Mux6/1 -> [RphiANDdphiAnkle]
  [RAnkleMoment] -> Multiply/1  "Torque"
  PS-Simulink Converter2/1 -> Rgiht Ankle Angle Torque/1, Mux6/1  "Angle"
  Otto-bock 3R60/1 -> To Workspace7/1, Mux5/1
  Otto-bock 3R60/2 -> Mux5/2
  Otto-bock 3R60/4 -> To Workspace1/1
  Otto-bock 3R60/5 -> To Workspace2/1
  Otto-bock 3R60/6 -> To Workspace4/1
  Otto-bock 3R60/7 -> To Workspace5/1
  Otto-bock 3R60/8 -> To Workspace6/1
  Multiply/1 -> Rgiht Ankle Angle Torque/2, Simulink-PS Converter1/1
  connections:
  TO: X-forward Y-up Z-lateral/RConn1 -- Mechanism Configuration/RConn1 -- Rigid Transform/LConn1 -- World Frame X-forward Y-lateral Z-up/RConn1 -- Solver Configuration/RConn1
  Left Ankle/RConn1 -- Left Shank/LConn1
  Left Ankle/RConn2 -- PS-Simulink Converter/LConn1
  Left Ankle/RConn3 -- PS-Simulink Converter1/LConn1
  Left Thigh/LConn1 -- Left Knee/RConn1
  Left Ankle/LConn2 -- Simulink-PS Converter/RConn1
  Simulink-PS Converter3/RConn1 -- Left Knee/LConn2
  Left Knee/RConn2 -- PS-Simulink Converter6/LConn1
  Left Knee/RConn3 -- PS-Simulink Converter7/LConn1
  Simulink-PS Converter4/RConn1 -- Left Hip/LConn2
  Left Hip/RConn2 -- PS-Simulink Converter8/LConn1
  Left Hip/RConn3 -- PS-Simulink Converter9/LConn1
  Rigid Transform/RConn1 -- Ground/RConn1
  Sensor Sheet/RConn1 -- Left Hip/LConn1
  Left Thigh/RConn1 -- Sensor Sheet/LConn1
  Thigh/RConn1 -- Amputated Thigh 3R60/RConn1 -- Sensor Sheet1/LConn1
  Right Hip/LConn1 -- Sensor Sheet1/RConn1
  Right Hip/LConn2 -- Simulink-PS Converter5/RConn1
  Right Hip/RConn3 -- PS-Simulink Converter11/LConn1
  Right Hip/RConn2 -- PS-Simulink Converter10/LConn1
  R Knee B Pos/Rot Sensor/LConn1 -- Amputated Thigh 3R60/LConn1 -- Thigh/LConn1 -- Rigid Transform/LConn1
  Ground Contact Model 2DNew2/LConn1 -- Right Foot/LConn2 -- R Ball Position Sensor/LConn1
  Left Hip/RConn1 -- L Hip Position Sensor/LConn1 -- Left Leg Angle/Length/LConn1 -- Rigid Transform2/LConn1 -- HAT/LConn1
  HAT/LConn2 -- Hip Pos/Speed Sensor/LConn1 -- Right Leg Angle/Length/LConn1 -- R Hip Position Sensor/LConn1 -- Right Hip/RConn1
  Left Knee/LConn1 -- L Knee Position Sensor/LConn1 -- Left Shank/RConn1
  Left Foot/LConn1 -- Ground Contact Model 2DNew4/LConn1 -- L Heel Position Sensor/LConn1
  Left Foot/LConn2 -- Planar Joint/RConn1 -- Ground Contact Model 2DNew1/LConn1 -- L Ball Position Sensor/LConn1
  HATTop Position Sensor/LConn1 -- HAT/RConn1
  Left Ankle/LConn1 -- Left Leg Angle/Length/LConn2 -- L Ankle Position Sensor/LConn1 -- Left Foot/RConn1
  R Knee B Pos/Rot Sensor/RConn1 -- Planar Joint/LConn1 -- TO: X-forward Y-up Z-lateral/LConn1 -- R Knee F Pos/Rot Sensor/RConn1
  HAT/RConn2 -- HAT Speed Sensor/LConn1 -- HAT Position Sensor/LConn1
  Right Leg Angle/Length/LConn2 -- Right Foot/LConn1 -- R Heel Position Sensor/LConn1 -- Ground Contact Model 2DNew3/LConn1
  L Shank Position Sensor/LConn1 -- Left Shank/LConn2
  Right Ankle/LConn1 -- R Ankle Position Sensor/LConn1 -- Right Foot/RConn1
  Right Ankle/RConn2 -- PS-Simulink Converter2/LConn1
  Right Ankle/LConn2 -- Simulink-PS Converter1/RConn1
  Prosthetic Shank/LConn1 -- Right Ankle/RConn1
  Right Ankle/RConn3 -- PS-Simulink Converter3/LConn1
  Rigid Transform1/LConn1 -- Rigid Transform3/LConn1 -- Otto-bock 3R60/RConn1
  Rigid Transform/RConn1 -- Otto-bock 3R60/LConn1
  Prosthetic Shank/RConn1 -- Rigid Transform1/RConn1
  Whole Body Tracking Camera/RConn1 -- Rigid Transform2/RConn1
  Prosthesis Tracking Camera/RConn1 -- Rigid Transform4/RConn1
  Rigid Transform4/LConn1 -- Rigid Transform3/RConn1

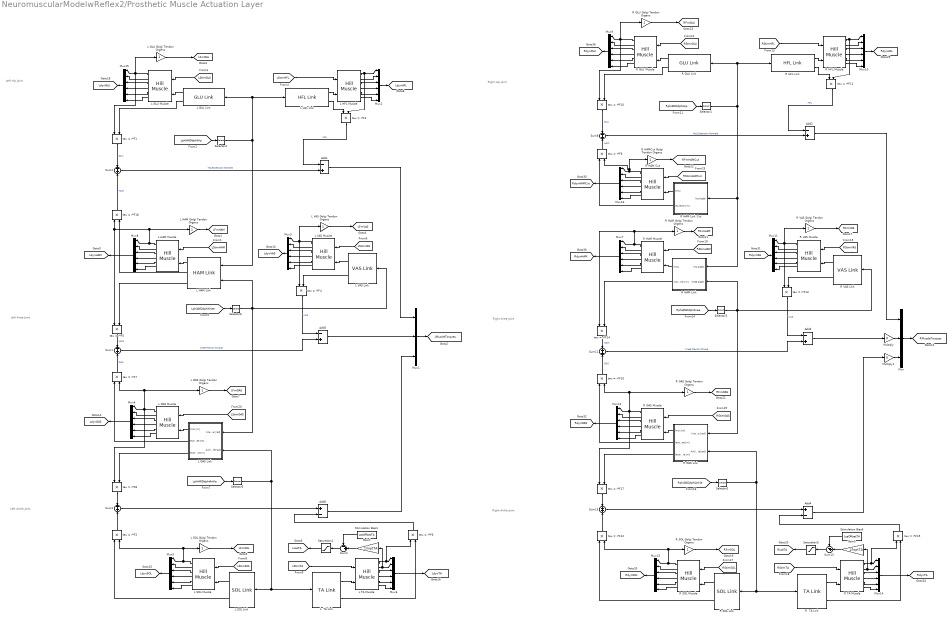
== system NeuromuscularModelwReflex2/Prosthetic Muscle Actuation Layer ==
  note: Right Hip Joint
  note: Right Knee Joint
  note: Right Ankle Joint
  note: Left Hip Joint
  note: Left Knee Joint
  note: Left Ankle Joint
  Add{1..3,5} (4 alike) : Sum  Inputs=-+
  Add4 : Sum  Inputs=+-
  Add6 : Sum  Inputs=+-
  Gain1 : Gain  Gain=1/loptTA
  Gain5 : Gain  Gain=1/loptTA
  L  TA Link : NeuroMuscularLibrary/TA Link  SystemSampleTime=-1  Latency=0  AutoFrameSizeCalculation=off
  L GAS Golgi Tendon Organs : Gain
  L GAS Link : Subsystem
  L GAS Muscle : NeuroMuscularLibrary/Hill Muscle  Fmax=FmaxGAS  lopt=loptGAS  vmax=vmaxGAS  lslack=lslackGAS
  L GLU Golgi Tendon Organs : Gain
  L GLU Link : NeuroMuscularLibrary/GLU Link  SystemSampleTime=-1  Latency=0  AutoFrameSizeCalculation=off
  L GLU Muscle : NeuroMuscularLibrary/Hill Muscle  Fmax=FmaxGLU  lopt=loptGLU  vmax=vmaxGLU  lslack=lslackGLU
  L HAM Golgi Tendon Organs : Gain
  L HAM Link : NeuroMuscularLibrary/HAM Link  SystemSampleTime=-1  Latency=0  AutoFrameSizeCalculation=off
  L HAM Muscle : NeuroMuscularLibrary/Hill Muscle  Fmax=FmaxHAM  lopt=loptHAM  vmax=vmaxHAM  lslack=lslackHAM
  L HFL Link : NeuroMuscularLibrary/HFL Link  SystemSampleTime=-1  Latency=0  AutoFrameSizeCalculation=off
  L HFL Muscle : NeuroMuscularLibrary/Hill Muscle  Fmax=FmaxHFL  lopt=loptHFL  vmax=vmaxHFL  lslack=lslackHFL
  L SOL Golgi Tendon Organs : Gain
  L SOL Link : NeuroMuscularLibrary/SOL Link  SystemSampleTime=-1  Latency=0  AutoFrameSizeCalculation=off
  L SOL Muscle : NeuroMuscularLibrary/Hill Muscle  Fmax=FmaxSOL  lopt=loptSOL  vmax=vmaxSOL  lslack=lslackSOL
  L TA Muscle : NeuroMuscularLibrary/Hill Muscle  Fmax=FmaxTA  lopt=loptTA  vmax=vmaxTA  lslack=lslackTA
  L VAS Golgi Tendon Organs : Gain
  L VAS Link : NeuroMuscularLibrary/VAS Link  SystemSampleTime=-1  Latency=0  AutoFrameSizeCalculation=off
  L VAS Muscle : NeuroMuscularLibrary/Hill Muscle  Fmax=FmaxVAS  lopt=loptVAS  vmax=vmaxVAS  lslack=lslackVAS
  Multiply : Gain  Gain=0
  Multiply1 : Gain  Gain=0
  Mux : Mux  Inputs=3
  Mux1 : Mux  Inputs=3
  Mux{2..16} (15 alike) : Mux  Inputs=6
  R  TA Link : NeuroMuscularLibrary/TA Link  SystemSampleTime=-1  Latency=0  AutoFrameSizeCalculation=off
  R GAS Golgi Tendon Organs : Gain
  R GAS Link : Subsystem
  R GAS Muscle : NeuroMuscularLibrary/Hill Muscle  Fmax=FmaxGAS  lopt=loptGAS  vmax=vmaxGAS  lslack=lslackGAS
  R GLU Golgi Tendon Organs : Gain
  R GLU Link : NeuroMuscularLibrary/GLU Link  SystemSampleTime=-1  Latency=0  AutoFrameSizeCalculation=off
  R GLU Muscle : NeuroMuscularLibrary/Hill Muscle  Fmax=FmaxGLU  lopt=loptGLU  vmax=vmaxGLU  lslack=lslackGLU
  R HAM Cut : NeuroMuscularLibrary/Hill Muscle  Fmax=FmaxHAMCut  lopt=loptHAMCut  vmax=vmaxHAM  lslack=lslackHAMCut
  R HAM Golgi Tendon Organs : Gain
  R HAM Link : Subsystem
  R HAM Link Cut : Subsystem
  R HAM Muscle : NeuroMuscularLibrary/Hill Muscle  Fmax=FmaxHAM  lopt=loptHAM  vmax=vmaxHAM  lslack=lslackHAM
  R HAMCut Golgi Tendon Organs : Gain
  R HFL Link : NeuroMuscularLibrary/HFL Link  SystemSampleTime=-1  Latency=0  AutoFrameSizeCalculation=off
  R HFL Muscle : NeuroMuscularLibrary/Hill Muscle  Fmax=FmaxHFL  lopt=loptHFL  vmax=vmaxHFL  lslack=lslackHFL
  R SOL Golgi Tendon Organs : Gain
  R SOL Link : NeuroMuscularLibrary/SOL Link  SystemSampleTime=-1  Latency=0  AutoFrameSizeCalculation=off
  R SOL Muscle : NeuroMuscularLibrary/Hill Muscle  Fmax=FmaxSOL  lopt=loptSOL  vmax=vmaxSOL  lslack=lslackSOL
  R TA Muscle : NeuroMuscularLibrary/Hill Muscle  Fmax=FmaxTA  lopt=loptTA  vmax=vmaxTA  lslack=lslackTA
  R VAS Golgi Tendon Organs : Gain
  R VAS Link : NeuroMuscularLibrary/VAS Link  SystemSampleTime=-1  Latency=0  AutoFrameSizeCalculation=off
  R VAS Muscle : NeuroMuscularLibrary/Hill Muscle  Fmax=FmaxVAS  lopt=loptVAS  vmax=vmaxVAS  lslack=lslackVAS
  Saturation1 : Saturate  UpperLimit=inf  LowerLimit=0
  Saturation5 : Saturate  UpperLimit=inf  LowerLimit=0
  Selector{1..6} (6 alike) : Selector  InputPortWidth=2  IndexOptions=Index vector (dialog)  Indices=1  OutputSizes=1
  Stimulation Bias1 : Constant  Value=LceOffsetTA
  Stimulation Bias6 : Constant  Value=LceOffsetTA
  Sum{1,3..4,8,11,15} (6 alike) : Sum  Inputs=+|+
  Sum13 : Sum  Inputs=-+|
  Sum2 : Sum  Inputs=-+|
  tau = r*F{1..18} (18 alike) : Product
  tag scope: LFmGAS=global, LFmGLU=global, LFmHAM=global, LFmSOL=global, LFmVAS=global, LLceTA=global, LMuscleTorques=global, LdynGAS=global, LdynGLU=global, LdynHAM=global, LdynHFL=global, LdynSOL=global, LdynTA=global, LdynVAS=global, RFmGAS=global, RFmGLU=global, RFmHAM=global, RFmHAMCut=global, RFmSOL=global, RFmVAS=global, RLceTA=global, RMuscleTorques=global, RdynGAS=global, RdynGLU=global, RdynHAM=global, RdynHAMCut=global, RdynHFL=global, RdynSOL=global, RdynTA=global, RdynVAS=global
  wires:
  R HAM Link/1(lmtu) -> R HAM Muscle/2
  R HAM Muscle/5 -> Mux7/5
  Mux7/1 -> [RdynHAM]
  R HAM Muscle/3 -> Mux7/3
  R HAM Muscle/4 -> Mux7/4
  [RphiANDdphiHip] -> Selector1/1
  Add2/1 -> Mux/1
  R GLU Link/1 -> R GLU Muscle/2
  [RStimGLU] -> R GLU Muscle/1
  R GLU Muscle/5 -> Mux9/5
  R GLU Muscle/2 -> Mux9/2
  R GLU Muscle/3 -> Mux9/3
  R GLU Muscle/4 -> Mux9/4
  R GLU Link/2 -> tau = r*F10/2
  R GLU Muscle/1 -> Mux9/1, R GLU Golgi Tendon Organs/1, tau = r*F10/1
  R GLU Golgi Tendon Organs/1 -> [RFmGLU]
  R HFL Link/1 -> R HFL Muscle/2
  [RStimHFL] -> R HFL Muscle/1
  R HFL Muscle/2 -> Mux10/2
  R HFL Muscle/5 -> Mux10/5
  Mux10/1 -> [RdynHFL]
  R HFL Muscle/4 -> Mux10/4
  R HFL Muscle/3 -> Mux10/3
  R HFL Link/2 -> tau = r*F11/1
  R HFL Muscle/1 -> Mux10/1, tau = r*F11/2
  R HAM Muscle/2 -> Mux7/2
  R HAM Golgi Tendon Organs/1 -> [RFmHAM]
  [RStimHAM] -> R HAM Muscle/1
  Add3/1 -> Multiply/1
  R VAS Link/1 -> R VAS Muscle/2
  R VAS Muscle/5 -> Mux11/5
  Mux11/1 -> [RdynVAS]
  R VAS Muscle/2 -> Mux11/2
  R VAS Muscle/3 -> Mux11/3
  R VAS Muscle/4 -> Mux11/4
  R VAS Muscle/1 -> R VAS Golgi Tendon Organs/1, Mux11/1, tau = r*F13/1
  R VAS Golgi Tendon Organs/1 -> [RFmVAS]
  R VAS Link/2 -> tau = r*F13/2
  R HAM Link/2(knee lever [m]) -> tau = r*F14/2
  Sum11/1 -> Add3/2  "Knee Flexion Torque"
  [RStimVAS] -> R VAS Muscle/1
  [RphiANDdphiKnee] -> Selector3/1
  R SOL Muscle/1 -> R SOL Golgi Tendon Organs/1, tau = r*F12/2, Mux13/1
  R SOL Muscle/5 -> Mux13/5
  Mux13/1 -> [RdynSOL]
  R SOL Muscle/2 -> Mux13/2
  R SOL Muscle/3 -> Mux13/3
  R SOL Muscle/4 -> Mux13/4
  R SOL Link/2 -> tau = r*F12/1
  R SOL Link/1 -> R SOL Muscle/2
  R SOL Golgi Tendon Organs/1 -> [RFmSOL]
  [RStimSOL] -> R SOL Muscle/1
  Selector2/1 -> R  TA Link/1, R SOL Link/1, R GAS Link/2(Ankle Angle[rad])
  [RphiANDdphiAnkle] -> Selector2/1
  Add4/1 -> Multiply1/1
  R  TA Link/1 -> R TA Muscle/2
  R TA Muscle/1 -> tau = r*F15/1, Mux14/1
  R TA Muscle/5 -> Mux14/5
  Mux14/1 -> [RdynTA]
  R TA Muscle/4 -> Mux14/4
  R TA Muscle/3 -> Mux14/3
  Sum13/1 -> Saturation5/1
  Saturation5/1 -> [RLceTA]
  [RStimTA] -> R TA Muscle/1
  Gain5/1 -> Sum13/2
  Stimulation Bias6/1 -> Sum13/1
  R  TA Link/2 -> tau = r*F15/2
  tau = r*F15/1 -> Add4/2
  R GAS Link/1(lmtu [m]) -> R GAS Muscle/2
  Selector3/1 -> R HAM Link/2(knee angle), R VAS Link/1, R GAS Link/1(Knee Angle [rad])
  R GAS Muscle/5 -> Mux12/5
  Mux12/1 -> [RdynGAS]
  R GAS Muscle/2 -> Mux12/2
  R GAS Muscle/3 -> Mux12/3
  R GAS Muscle/4 -> Mux12/4
  R GAS Link/2(leverKnee [m]) -> tau = r*F16/1
  [RStimGAS] -> R GAS Muscle/1
  tau = r*F12/1 -> Sum15/2
  Sum15/1 -> Add4/1
  R GAS Link/3(leverAnkle [m]) -> tau = r*F17/2
  tau = r*F17/1 -> Sum15/1
  R GAS Muscle/1 -> Mux12/1, tau = r*F16/2, R GAS Golgi Tendon Organs/1, tau = r*F17/1
  R GAS Golgi Tendon Organs/1 -> [RFmGAS]
  tau = r*F9/1 -> Sum8/2  "HAM"
  tau = r*F10/1 -> Sum8/1  "GLU"
  tau = r*F11/1 -> Add2/1  "HFL"
  R HAM Muscle/1 -> tau = r*F14/1, R HAM Golgi Tendon Organs/1, Mux7/1
  Sum8/1 -> Add2/2  "Hip Extension Moment"
  tau = r*F16/1 -> Sum11/2  "GAS"
  tau = r*F14/1 -> Sum11/1  "HAM"
  tau = r*F13/1 -> Add3/1  "VAS"
  R TA Muscle/2 -> Gain5/1, Mux14/2
  Mux9/1 -> [RdynGLU]
  Mux/1 -> [RMuscleTorques]
  L HAM Link/1 -> L HAM Muscle/2
  L HAM Link/2 -> tau = r*F18/2
  L HAM Muscle/5 -> Mux8/5
  Mux8/1 -> [LdynHAM]
  L HAM Muscle/3 -> Mux8/3
  L HAM Muscle/4 -> Mux8/4
  [LphiANDdphiHip] -> Selector4/1
  Selector4/1 -> L HAM Link/1, L GLU Link/1, L HFL Link/1
  Add1/1 -> Mux1/1
  L GLU Link/1 -> L GLU Muscle/2
  [LStimGLU] -> L GLU Muscle/1
  L GLU Muscle/5 -> Mux15/5
  L GLU Muscle/2 -> Mux15/2
  L GLU Muscle/3 -> Mux15/3
  L GLU Muscle/4 -> Mux15/4
  L GLU Link/2 -> tau = r*F1/2
  L GLU Muscle/1 -> Mux15/1, L GLU Golgi Tendon Organs/1, tau = r*F1/1
  L GLU Golgi Tendon Organs/1 -> [LFmGLU]
  L HFL Link/1 -> L HFL Muscle/2
  [LStimHFL] -> L HFL Muscle/1
  L HFL Muscle/2 -> Mux2/2
  L HFL Muscle/5 -> Mux2/5
  Mux2/1 -> [LdynHFL]
  L HFL Muscle/4 -> Mux2/4
  L HFL Muscle/3 -> Mux2/3
  L HFL Link/2 -> tau = r*F2/1
  L HFL Muscle/1 -> Mux2/1, tau = r*F2/2
  L HAM Muscle/2 -> Mux8/2
  L HAM Golgi Tendon Organs/1 -> [LFmHAM]
  [LStimHAM] -> L HAM Muscle/1
  Add5/1 -> Mux1/2
  L VAS Link/1 -> L VAS Muscle/2
  L VAS Muscle/5 -> Mux3/5
  Mux3/1 -> [LdynVAS]
  L VAS Muscle/2 -> Mux3/2
  L VAS Muscle/3 -> Mux3/3
  L VAS Muscle/4 -> Mux3/4
  L VAS Muscle/1 -> L VAS Golgi Tendon Organs/1, Mux3/1, tau = r*F4/1
  L VAS Golgi Tendon Organs/1 -> [LFmVAS]
  L VAS Link/2 -> tau = r*F4/2
  L HAM Link/3 -> tau = r*F5/2
  Sum1/1 -> Add5/2  "Knee Flexion Torque"
  [LStimVAS] -> L VAS Muscle/1
  [LphiANDdphiKnee] -> Selector6/1
  L SOL Muscle/1 -> L SOL Golgi Tendon Organs/1, tau = r*F3/2, Mux5/1
  L SOL Muscle/5 -> Mux5/5
  Mux5/1 -> [LdynSOL]
  L SOL Muscle/2 -> Mux5/2
  L SOL Muscle/3 -> Mux5/3
  L SOL Muscle/4 -> Mux5/4
  L SOL Link/2 -> tau = r*F3/1
  L SOL Link/1 -> L SOL Muscle/2
  L SOL Golgi Tendon Organs/1 -> [LFmSOL]
  [LStimSOL] -> L SOL Muscle/1
  Selector5/1 -> L  TA Link/1, L SOL Link/1, L GAS Link/2(Ankle Angle[rad])
  [LphiANDdphiAnkle] -> Selector5/1
  Add6/1 -> Mux1/3
  L  TA Link/1 -> L TA Muscle/2
  L TA Muscle/1 -> tau = r*F6/1, Mux6/1
  L TA Muscle/5 -> Mux6/5
  Mux6/1 -> [LdynTA]
  L TA Muscle/4 -> Mux6/4
  L TA Muscle/3 -> Mux6/3
  Sum2/1 -> Saturation1/1
  Saturation1/1 -> [LLceTA]
  [LStimTA] -> L TA Muscle/1
  Gain1/1 -> Sum2/2
  Stimulation Bias1/1 -> Sum2/1
  L  TA Link/2 -> tau = r*F6/2
  tau = r*F6/1 -> Add6/2
  L GAS Link/1(lmtu [m]) -> L GAS Muscle/2
  Selector6/1 -> L HAM Link/2, L VAS Link/1, L GAS Link/1(Knee Angle [rad])
  L GAS Muscle/5 -> Mux4/5
  Mux4/1 -> [LdynGAS]
  L GAS Muscle/2 -> Mux4/2
  L GAS Muscle/3 -> Mux4/3
  L GAS Muscle/4 -> Mux4/4
  L GAS Link/2(leverKnee [m]) -> tau = r*F7/1
  [LStimGAS] -> L GAS Muscle/1
  tau = r*F3/1 -> Sum3/2
  Sum3/1 -> Add6/1
  L GAS Link/3(leverAnkle [m]) -> tau = r*F8/2
  tau = r*F8/1 -> Sum3/1
  L GAS Muscle/1 -> Mux4/1, tau = r*F7/2, L GAS Golgi Tendon Organs/1, tau = r*F8/1
  L GAS Golgi Tendon Organs/1 -> [LFmGAS]
  tau = r*F18/1 -> Sum4/2  "HAM"
  tau = r*F1/1 -> Sum4/1  "GLU"
  tau = r*F2/1 -> Add1/1  "HFL"
  L HAM Muscle/1 -> tau = r*F5/1, tau = r*F18/1, L HAM Golgi Tendon Organs/1, Mux8/1
  Sum4/1 -> Add1/2  "Hip Extension Moment"
  tau = r*F7/1 -> Sum1/2  "GAS"
  tau = r*F5/1 -> Sum1/1  "HAM"
  tau = r*F4/1 -> Add5/1  "VAS"
  L TA Muscle/2 -> Gain1/1, Mux6/2
  Mux15/1 -> [LdynGLU]
  Mux1/1 -> [LMuscleTorques]
  Selector1/1 -> R HAM Link/1(hip angle), R HAM Link Cut/1(hip angle), R GLU Link/1, R HFL Link/1
  R HAM Cut/5 -> Mux16/5
  R HAM Cut/3 -> Mux16/3
  R HAM Cut/4 -> Mux16/4
  R HAM Cut/2 -> Mux16/2
  R HAM Cut/1 -> Mux16/1, tau = r*F9/2, R HAMCut Golgi Tendon Organs/1
  [RStimHAMCut] -> R HAM Cut/1
  R HAM Link Cut/1(lmtu) -> R HAM Cut/2
  R HAM Link Cut/2(hip lever [m]) -> tau = r*F9/1
  Mux16/1 -> [RdynHAMCut]
  R HAMCut Golgi Tendon Organs/1 -> [RFmHAMCut]
  Multiply/1 -> Mux/2
  Multiply1/1 -> Mux/3
  L GLU Muscle/6 -> Mux15/6
  L HFL Muscle/6 -> Mux2/6
  L HAM Muscle/6 -> Mux8/6
  L VAS Muscle/6 -> Mux3/6
  L GAS Muscle/6 -> Mux4/6
  L SOL Muscle/6 -> Mux5/6
  L TA Muscle/6 -> Mux6/6
  R GLU Muscle/6 -> Mux9/6
  R HFL Muscle/6 -> Mux10/6
  R HAM Cut/6 -> Mux16/6
  R HAM Muscle/6 -> Mux7/6
  R VAS Muscle/6 -> Mux11/6
  R GAS Muscle/6 -> Mux12/6
  R SOL Muscle/6 -> Mux13/6
  R TA Muscle/6 -> Mux14/6
